simulink model "STH3b1"  (R2021b)
settings: Solver=VariableStepAuto  StartTime=0.0  StopTime=1800  FixedStep=1  RelTol=1e-3
values from neighbouring files (symbols this model uses):
  dF = 0    [main_exp4.m]
  dTi = 0    [main_exp4.m]
  dTij = 0    [main_exp4.m]
  Fjs = 7.079e-4    (= 0.0007079)    [main_exp4.m]
  Fs = 4.720e-4    (= 0.000472)    [main_exp4.m]
  kp_simc3a1 = T11p1/(G011p1*(taoc_3a1 + L11p1))    (= 5.03711849265)    [main_exp4.m]
  RefT = 53.67    [main_exp4.m]
  Ti_simc3a1 = min(T11p1, 4*(taoc_3a1 + L11p1))    [main_exp4.m]
  Tis = 10    [main_exp4.m]
  Tjis = 93.33    [main_exp4.m]
  Tjs = 65.56    [main_exp4.m]
  Ts = 51.67    [main_exp4.m]
libraries: slpidlib x1
settings Model: Creator=luang  LastModifiedBy=luang

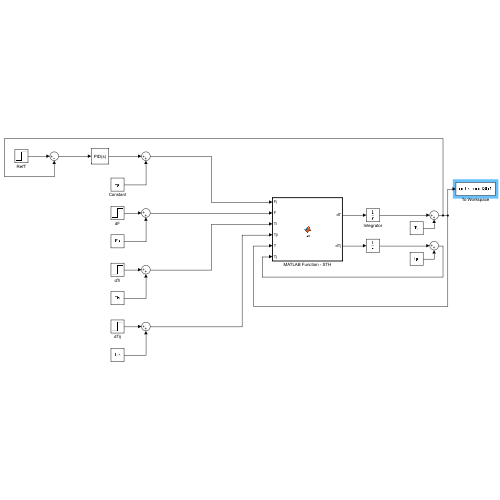
[thumbnail: Simulink's stored preview of the top-level diagram]
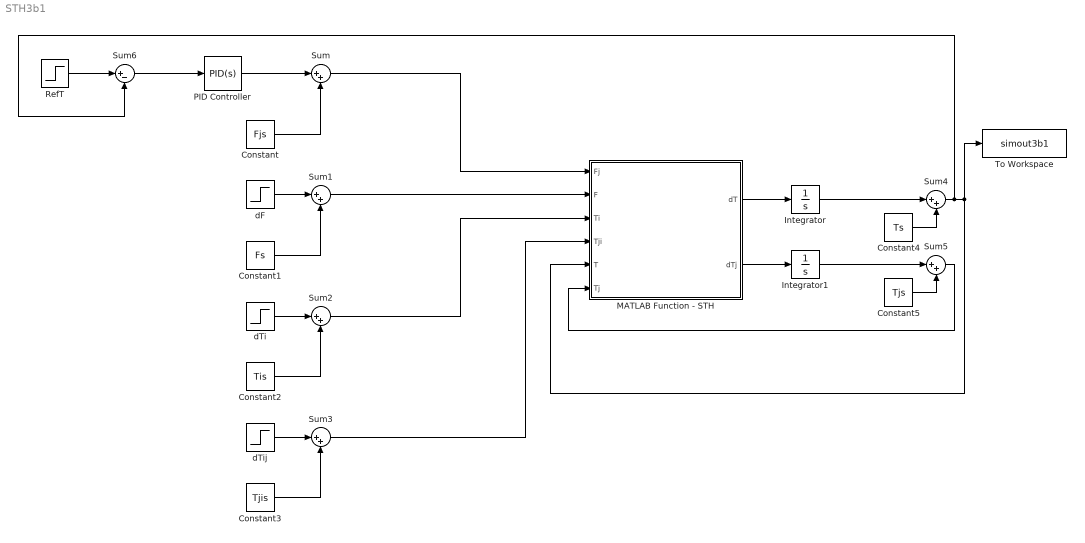
== system STH3b1 ==
  Constant : Constant  Value=Fjs
  Constant1 : Constant  Value=Fs
  Constant2 : Constant  Value=Tis
  Constant3 : Constant  Value=Tjis
  Constant4 : Constant  Value=Ts
  Constant5 : Constant  Value=Tjs
  Integrator : Integrator
  Integrator1 : Integrator
  MATLAB Function - STH : MATLAB Function  TreatAsAtomicUnit=on
  PID Controller : slpidlib/PID Controller  Controller=PID  Form=Parallel  TimeDomain=Continuous-time  UseExternalTs=off  SampleTime=-1  IntegratorMethod=Forward Euler  FilterMethod=Forward Euler  ControllerParametersSource=internal  P=kp_simc3a1  I=kp_simc3a1/Ti_simc3a1  D=0  UseFilter=on  N=100  TunerSelectOption=Transfer Function Based (PID Tuner App)  InitialConditionSource=internal  InitialConditionForIntegrator=0  InitialConditionForFilter=0  DifferentiatorICPrevScaledInput=0  ExternalReset=none  TrackingMode=off  Kt=1  LimitOutput=off  SatLimitsSource=internal  UpperSaturationLimit=inf  LowerSaturationLimit=-inf  LinearizeAsGain=on  AntiWindupMode=none  Kb=1  POutMin=[]  POutMax=[]  IOutMin=[]  IOutMax=[]  DOutMin=[]  DOutMax=[]  NOutMin=[]  NOutMax=[]  SumOutMin=[]  SumOutMax=[]  SaturationOutMin=[]  SaturationOutMax=[]  PParamMin=[]  PParamMax=[]  IParamMin=[]  IParamMax=[]  DParamMin=[]  DParamMax=[]  NParamMin=[]  NParamMax=[]  KbParamMin=[]  KbParamMax=[]  KtParamMin=[]  KtParamMax=[]  KbOutMin=[]  KbOutMax=[]  KtOutMin=[]  KtOutMax=[]  IntegratorOutMin=[]  IntegratorOutMax=[]  FilterOutMin=[]  FilterOutMax=[]  SumI1OutMin=[]  SumI1OutMax=[]  SumI2OutMin=[]  SumI2OutMax=[]  SumI3OutMin=[]  SumI3OutMax=[]  SumI4OutMin=[]  SumI4OutMax=[]  SumDOutMin=[]  SumDOutMax=[]  DifferentiatorOutMin=[]  DifferentiatorOutMax=[]  FilterDiffOutCoefMin=[]  FilterDiffOutCoefMax=[]  ReciprocalOutMin=[]  ReciprocalOutMax=[]  SumDenOutMin=[]  SumDenOutMax=[]  SumNumOutMin=[]  SumNumOutMax=[]  DivideOutMin=[]  DivideOutMax=[]  UdiffTsProdOutMin=[]  UdiffTsProdOutMax=[]  NTsProdOutMin=[]  NTsProdOutMax=[]  UintegralTsProdOutMin=[]  UintegralTsProdOutMax=[]  UngainTsProdOutMin=[]  UngainTsProdOutMax=[]  IntegratorContinuousStateAttributes=''  IntegratorStateMustResolveToSignalObject=off  IntegratorRTWStateStorageClass=Auto  FilterContinuousStateAttributes=''  FilterStateMustResolveToSignalObject=off  FilterRTWStateStorageClass=Auto  ParallelPVariant=InternalParameters  IdealPVariant=Disabled  IVariant=InternalParameters  DVariant=InternalParameters  IntegratorVariant=Continuous  SatVariant=Disabled  AWVariant=Passthrough  PCopyVariant=Disabled  TRVariant=Disabled  FdbkBlocksVariant=Forward  IdealPFdbkVariant=Disabled  SatFdbkVariant=Disabled  DerivativeFilterVariant=ContFilter  NVariant=InternalParameters  NCopyVariant=Disabled  FilterICVariant=InternalICsFilter  IntegratorICVariant=InternalICs  ExternalResetVariant=Disabled  TRSumVariant=Passthrough  SumFdbkVariant=Disabled  SumVariant=Sum_PID  TsampFilterVariant=InternalTs  TsampNgainVariant=Passthrough  TsampIntegralVariant=Passthrough  ExternalSaturationOutDataTypeStr=Inherit: Same as second input
  RefT : Step  Before=Ts  After=RefT  SampleTime=0
  Sum{,1..5} (6 alike) : Sum  Inputs=|++
  Sum6 : Sum  Inputs=|+-
  To Workspace : ToWorkspace  VariableName=simout3b1  SaveFormat=Structure With Time  SampleTime=-1
  dF : Step  After=dF  SampleTime=0
  dTi : Step  After=dTi  SampleTime=0
  dTij : Step  After=dTij  SampleTime=0
  wires:
  Constant/1 -> Sum/2
  Constant1/1 -> Sum1/2
  dF/1 -> Sum1/1
  Constant2/1 -> Sum2/2
  dTi/1 -> Sum2/1
  Constant3/1 -> Sum3/2
  dTij/1 -> Sum3/1
  Sum/1 -> MATLAB Function - STH/1(Fj)
  Sum1/1 -> MATLAB Function - STH/2(F)
  Sum2/1 -> MATLAB Function - STH/3(Ti)
  Sum3/1 -> MATLAB Function - STH/4(Tji)
  MATLAB Function - STH/1(dT) -> Integrator/1
  MATLAB Function - STH/2(dTj) -> Integrator1/1
  Integrator/1 -> Sum4/1
  Constant4/1 -> Sum4/2
  Constant5/1 -> Sum5/2
  Integrator1/1 -> Sum5/1
  Sum4/1 -> Sum6/2, To Workspace/1, MATLAB Function - STH/5(T)
  Sum5/1 -> MATLAB Function - STH/6(Tj)
  RefT/1 -> Sum6/1
  Sum6/1 -> PID Controller/1
  PID Controller/1 -> Sum/1

== matlab function STH3b1/MATLAB Function - STH ==
  data: Fj input; dT output; F input; Ti input; Tji input; T input; Tj input; dTj output
function [dT, dTj] = fcn(Fj, F, Ti, Tji, T, Tj)

V = 283.168e-3;
UA = 3.065;
pcp = 2.165e3;
Vj = 28.319e-3;
pcpj = 2.165e3;

dT = (F/V)*(Ti - T) + (UA/(V*pcp))*(Tj - T);

dTj = (Fj/Vj)*(Tji - Tj) - ((UA/(Vj*pcpj))*(Tj - T));
